simulink model "nsdynamic"  (Simulink 9.0)
settings: Solver=ode4  StartTime=0.0  StopTime=10.0  FixedStep=0.01  RelTol=1e-3
InitFcn:
  | iniNS
settings Model: Creator=ABDULJAWAD KAYALI  LastModifiedBy=ABDULJAWAD KAYALI
settings DataIOCC: SaveFormat=Dataset
settings OptimizationCC: LifeSpan=auto
settings DebuggingCC: UnderspecifiedInitializationDetection=Simplified  MergeDetectMultiDrivingBlocksExec=error  SFUnexpectedBacktrackingDiag=error  SFNoUnconditionalDefaultTransitionDiag=error  SFExecutionAtInitializationDiag=warning
settings HardwareCC: ProdBitPerPointer=64  ProdBitPerSizeT=64  ProdBitPerPtrDiffT=64  ProdLargestAtomicFloat=Float  ProdIntDivRoundTo=Zero  ProdEndianess=LittleEndian  ProdWordSize=64  ProdHWDeviceType=Intel->x86-64 (Windows64)
settings ModelReferenceCC: PropagateSignalLabelsOutOfModel=on
settings CodeAppCC: StateflowObjectComments=off
settings GRTTargetCC: TargetLangStandard=C99 (ISO)
settings ConfigComp: CovMetricSettings=dwe  CovHtmlReporting=off  CovSaveCumulativeToWorkspaceVar=off  CovSaveSingleToWorkspaceVar=off  CovExternalEMLEnable=on

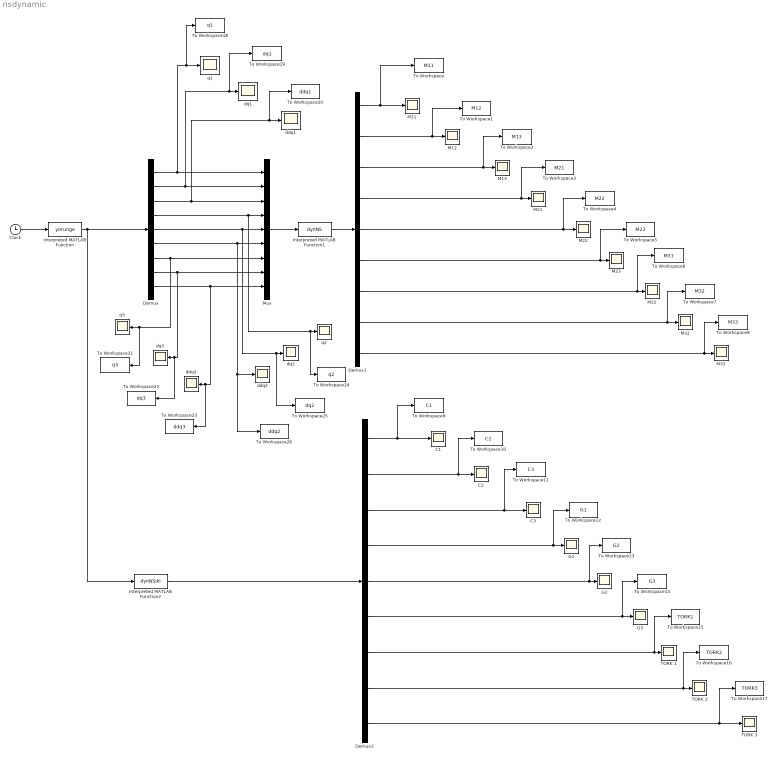
== system nsdynamic ==
  " TORK 1" : Scope
  "C1 " : Scope
  C2 : Scope
  C3 : Scope
  Clock : Clock
  Demux : Demux  Outputs=9
  Demux1 : Demux  Outputs=9
  Demux2 : Demux  Outputs=9
  G1 : Scope
  G2 : Scope
  G3 : Scope
  Interpreted MATLAB Function : MATLABFcn  MATLABFcn=yorunge
  Interpreted MATLAB Function1 : MATLABFcn  MATLABFcn=dynNS
  Interpreted MATLAB Function2 : MATLABFcn  MATLABFcn=dynNSiki
  M{11..13,21..23} (6 alike) : Scope
  "M31 " : Scope
  "M32 " : Scope
  "M33 " : Scope
  Mux : Mux  Inputs=9
  TORK 2 : Scope
  "TORK 3 " : Scope
  To Workspace : ToWorkspace  VariableName=M11  SaveFormat=Timeseries  SampleTime=-1
  To Workspace1 : ToWorkspace  VariableName=M12  SaveFormat=Timeseries  SampleTime=-1
  To Workspace10 : ToWorkspace  VariableName=C2  SaveFormat=Timeseries  SampleTime=-1
  To Workspace11 : ToWorkspace  VariableName=C3  SaveFormat=Timeseries  SampleTime=-1
  To Workspace12 : ToWorkspace  VariableName=G1  SaveFormat=Timeseries  SampleTime=-1
  To Workspace13 : ToWorkspace  VariableName=G2  SaveFormat=Timeseries  SampleTime=-1
  To Workspace14 : ToWorkspace  VariableName=G3  SaveFormat=Timeseries  SampleTime=-1
  To Workspace15 : ToWorkspace  VariableName=TORK1  SaveFormat=Timeseries  SampleTime=-1
  To Workspace16 : ToWorkspace  VariableName=TORK2  SaveFormat=Timeseries  SampleTime=-1
  To Workspace17 : ToWorkspace  VariableName=TORK3  SaveFormat=Timeseries  SampleTime=-1
  To Workspace18 : ToWorkspace  VariableName=q1  SaveFormat=Timeseries  SampleTime=-1
  To Workspace19 : ToWorkspace  VariableName=dq1  SaveFormat=Timeseries  SampleTime=-1
  To Workspace2 : ToWorkspace  VariableName=M13  SaveFormat=Timeseries  SampleTime=-1
  To Workspace20 : ToWorkspace  VariableName=ddq1  SaveFormat=Timeseries  SampleTime=-1
  To Workspace21 : ToWorkspace  VariableName=q3  SaveFormat=Timeseries  SampleTime=-1
  To Workspace22 : ToWorkspace  VariableName=dq3  SaveFormat=Timeseries  SampleTime=-1
  To Workspace23 : ToWorkspace  VariableName=ddq3  SaveFormat=Timeseries  SampleTime=-1
  To Workspace24 : ToWorkspace  VariableName=q2  SaveFormat=Timeseries  SampleTime=-1
  To Workspace25 : ToWorkspace  VariableName=dq2  SaveFormat=Timeseries  SampleTime=-1
  To Workspace26 : ToWorkspace  VariableName=ddq2  SaveFormat=Timeseries  SampleTime=-1
  To Workspace3 : ToWorkspace  VariableName=M21  SaveFormat=Timeseries  SampleTime=-1
  To Workspace4 : ToWorkspace  VariableName=M22  SaveFormat=Timeseries  SampleTime=-1
  To Workspace5 : ToWorkspace  VariableName=M23  SaveFormat=Timeseries  SampleTime=-1
  To Workspace6 : ToWorkspace  VariableName=M31  SaveFormat=Timeseries  SampleTime=-1
  To Workspace7 : ToWorkspace  VariableName=M32  SaveFormat=Timeseries  SampleTime=-1
  To Workspace8 : ToWorkspace  VariableName=M33  SaveFormat=Timeseries  SampleTime=-1
  To Workspace9 : ToWorkspace  VariableName=C1  SaveFormat=Timeseries  SampleTime=-1
  "ddq1 " : Scope
  "ddq2 " : Scope
  ddq3 : Scope
  "dq1 " : Scope
  "dq2 " : Scope
  dq3 : Scope
  "q1 " : Scope
  "q2 " : Scope
  "q3 " : Scope
  wires:
  Clock/1 -> Interpreted MATLAB Function/1
  Interpreted MATLAB Function/1 -> Demux/1, Interpreted MATLAB Function2/1
  Demux/1 -> To Workspace18/1, "q1 "/1, Mux/1
  Demux/2 -> To Workspace19/1, "dq1 "/1, Mux/2
  Demux/3 -> To Workspace20/1, "ddq1 "/1, Mux/3
  Demux/4 -> To Workspace24/1, "q2 "/1, Mux/4
  Demux/5 -> To Workspace25/1, "dq2 "/1, Mux/5
  Demux/6 -> "ddq2 "/1, To Workspace26/1, Mux/6
  Demux/7 -> To Workspace21/1, "q3 "/1, Mux/7
  Demux/8 -> To Workspace22/1, dq3/1, Mux/8
  Demux/9 -> To Workspace23/1, ddq3/1, Mux/9
  Demux1/2 -> To Workspace1/1, M12/1
  Demux1/3 -> To Workspace2/1, M13/1
  Demux1/4 -> To Workspace3/1, M21/1
  Demux1/5 -> To Workspace4/1, M22/1
  Demux1/6 -> To Workspace5/1, M23/1
  Demux1/7 -> To Workspace6/1, "M31 "/1
  Demux1/9 -> To Workspace8/1, "M33 "/1
  Mux/1 -> Interpreted MATLAB Function1/1
  Interpreted MATLAB Function1/1 -> Demux1/1
  Demux2/5 -> To Workspace13/1, G2/1
  Demux2/4 -> To Workspace12/1, G1/1
  Demux2/6 -> To Workspace14/1, G3/1
  Demux2/8 -> To Workspace16/1, TORK 2/1
  Demux2/2 -> To Workspace10/1, C2/1
  Demux2/1 -> To Workspace9/1, "C1 "/1
  Demux2/3 -> To Workspace11/1, C3/1
  Demux2/9 -> To Workspace17/1, "TORK 3 "/1
  Demux2/7 -> To Workspace15/1, " TORK 1"/1
  Interpreted MATLAB Function2/1 -> Demux2/1
  Demux1/1 -> To Workspace/1, M11/1
  Demux1/8 -> To Workspace7/1, "M32 "/1
